simulink model "missile_simulink"  (R2025a)
settings: Solver=ode4  StartTime=0.0  StopTime=300  FixedStep=0.01  RelTol=1e-3
values from neighbouring files (symbols this model uses):
  ka = 4.5    [missile_sim.m]
  kd = 1.1    [missile_sim.m]
  ki = 14.3    [missile_sim.m]
  kr = -0.37    [missile_sim.m]
  l_m0 = 40 * d2r    (= 0.698131700798)    [missile_sim.m]
  l_t0 = -2.5 * d2r    (= -0.0436332312999)    [missile_sim.m]
  v_t = 1000    [missile_sim.m]
  x_m0 = 2000    [missile_sim.m]
  x_t0 = 100    [missile_sim.m]
  z_m0 = 0    [missile_sim.m]
  z_t0 = 20000    [missile_sim.m]
libraries: simulink x1
settings Model: Creator=jWmma  LastModifiedBy=jWmma
settings DebuggingCC: SolverPrmCheckMsg=warning

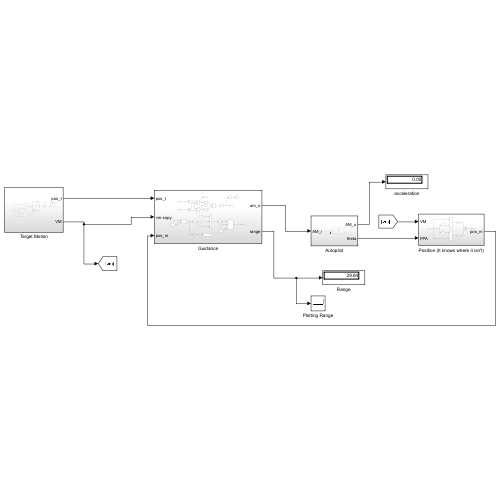
[thumbnail: Simulink's stored preview of the top-level diagram]
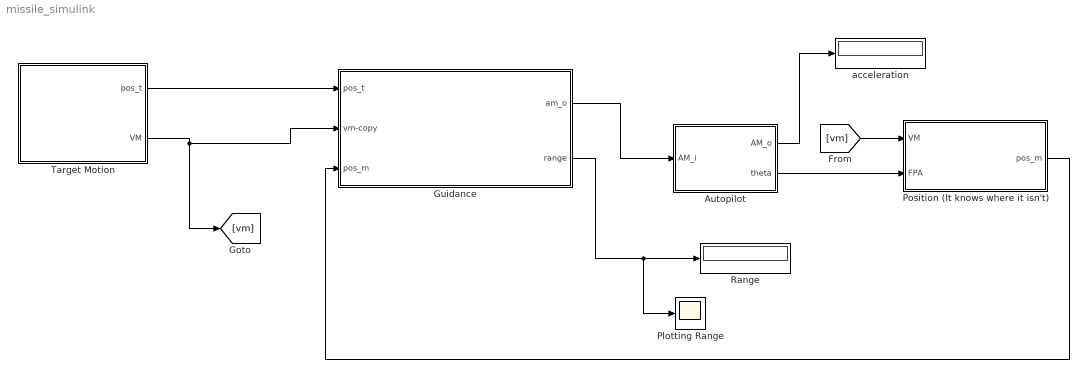
== system missile_simulink ==
  Autopilot : Subsystem
  Guidance : Subsystem
  Plotting Range : Scope
      settings: ActiveDisplayYMinimum=-88.233832620361682  ActiveDisplayYMaximum=93.627607111777422
  Position (It knows where it isn't) : Subsystem
  Range : Display
      settings: Format=bank
  Target Motion : Subsystem
  acceleration : Display
      settings: Format=bank
  wires:
  Guidance/1(am_o) -> Autopilot/1(AM_i)
  Guidance/2(range) -> Plotting Range/1, Range/1
  Autopilot/2(theta) -> Position (It knows where it isn't)/2(FPA)
  Position (It knows where it isn't)/1(pos_m) -> Guidance/3(pos_m)
  Target Motion/1(pos_t) -> Guidance/1(pos_t)
  Target Motion/2(VM) -> [vm], Guidance/2(vm-copy)
  Autopilot/1(AM_o) -> acceleration/1
  [vm] -> Position (It knows where it isn't)/1(VM)

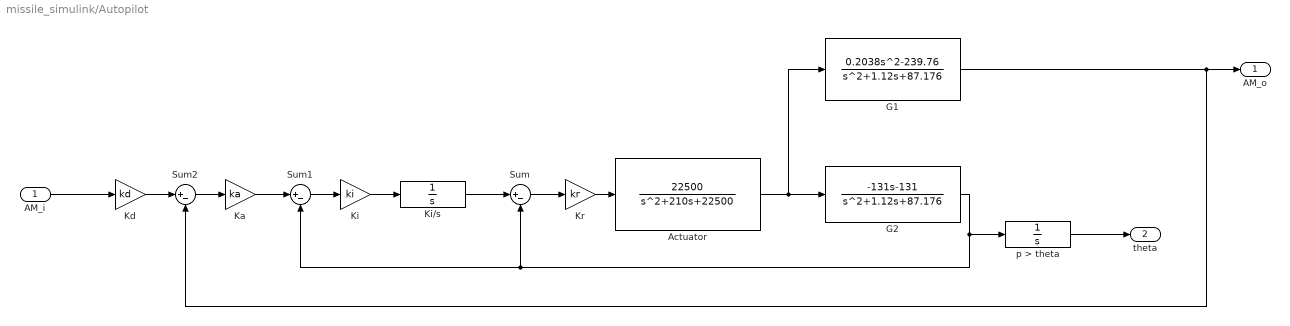
== system missile_simulink/Autopilot ==
  AM_i : Inport
  Actuator : TransferFcn  Numerator=[22500]  Denominator=[1 210 22500]
  G1 : TransferFcn  Numerator=[0.2038 0 -239.76]  Denominator=[1 1.12 87.176]
  G2 : TransferFcn  Numerator=[-131 -131]  Denominator=[1 1.12 87.176]
  Ka : Gain  Gain=ka
  Kd : Gain  Gain=kd
  Ki : Gain  Gain=ki
  Ki/s : Integrator
  Kr : Gain  Gain=kr
  Sum : Sum  Inputs=|+-
  Sum1 : Sum  Inputs=|+-
  Sum2 : Sum  Inputs=|+-
  p > theta : Integrator  InitialCondition=l_m0
  AM_o : Outport
  theta : Outport  Port=2
  wires:
  p > theta/1 -> theta/1
  Sum2/1 -> Ka/1
  G2/1 -> p > theta/1, Sum1/2, Sum/2
  AM_i/1 -> Kd/1
  Actuator/1 -> G1/1, G2/1
  Kr/1 -> Actuator/1
  Ka/1 -> Sum1/1
  Sum1/1 -> Ki/1
  Sum/1 -> Kr/1
  G1/1 -> AM_o/1, Sum2/2
  Ki/1 -> Ki/s/1
  Ki/s/1 -> Sum/1
  Kd/1 -> Sum2/1

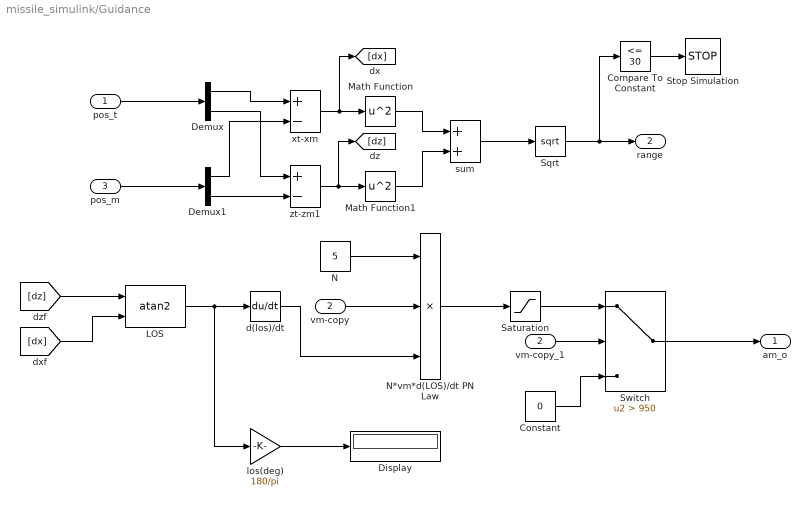
== system missile_simulink/Guidance ==
  pos_t : Inport
  vm-copy : Inport  Port=2
  pos_m : Inport  Port=3
  Compare To Constant : simulink/Logic and Bit Operations/Compare To Constant  relop=<=  const=30  OutDataTypeStr=boolean
  Constant : Constant  Value=0
  Demux : Demux  Outputs=2
  Demux1 : Demux  Outputs=2
  Display : Display
  LOS : Trigonometry  Operator=atan2
  Math Function : Math  Operator=square  OutputSignalType=real
  Math Function1 : Math  Operator=square  OutputSignalType=real
  N : Constant  Value=5
  N*vm*d(LOS)/dt PN Law : Product  Inputs=3
  Saturation : Saturate  UpperLimit=0  LowerLimit=-0.1
  Sqrt : Sqrt
  Stop Simulation : Stop
  Switch : Switch  Criteria=u2 > Threshold  Threshold=950  SaturateOnIntegerOverflow=off  InputSameDT=off
  d(los)/dt : Derivative
  los(deg) : Gain  Gain=180/pi
  sum : Sum
  vm-copy_1 : InportShadow  Port=2
  xt-xm : Sum  Inputs=+-
  zt-zm1 : Sum  Inputs=+-
  am_o : Outport
  range : Outport  Port=2
  wires:
  Math Function1/1 -> sum/2
  Demux1/2 -> zt-zm1/2
  N/1 -> N*vm*d(LOS)/dt PN Law/1
  vm-copy_1/1 -> Switch/2
  xt-xm/1 -> [dx], Math Function/1
  LOS/1 -> los(deg)/1, d(los)/dt/1
  Demux/2 -> zt-zm1/1
  zt-zm1/1 -> [dz], Math Function1/1
  Demux1/1 -> xt-xm/2
  [dx] -> LOS/2
  [dz] -> LOS/1
  los(deg)/1 -> Display/1
  pos_t/1 -> Demux/1
  Math Function/1 -> sum/1
  Sqrt/1 -> Compare To Constant/1, range/1
  vm-copy/1 -> N*vm*d(LOS)/dt PN Law/2
  pos_m/1 -> Demux1/1
  Demux/1 -> xt-xm/1
  sum/1 -> Sqrt/1
  Constant/1 -> Switch/3
  N*vm*d(LOS)/dt PN Law/1 -> Saturation/1
  d(los)/dt/1 -> N*vm*d(LOS)/dt PN Law/3
  Saturation/1 -> Switch/1
  Switch/1 -> am_o/1
  Compare To Constant/1 -> Stop Simulation/1

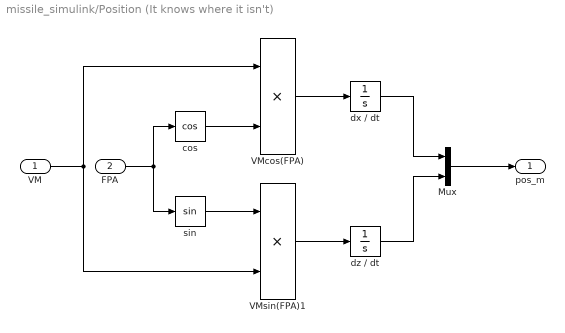
== system missile_simulink/Position (It knows where it isn't) ==
  VM : Inport
  FPA : Inport  Port=2
  Mux : Mux  Inputs=2
  VMcos(FPA) : Product
  VMsin(FPA)1 : Product
  cos : Trigonometry  Operator=cos
  dx / dt : Integrator  InitialCondition=x_m0
  dz / dt : Integrator  InitialCondition=z_m0
  sin : Trigonometry
  pos_m : Outport
  wires:
  VMsin(FPA)1/1 -> dz / dt/1
  VMcos(FPA)/1 -> dx / dt/1
  VM/1 -> VMsin(FPA)1/2, VMcos(FPA)/1
  Mux/1 -> pos_m/1
  dz / dt/1 -> Mux/2
  dx / dt/1 -> Mux/1
  sin/1 -> VMsin(FPA)1/1
  FPA/1 -> sin/1, cos/1
  cos/1 -> VMcos(FPA)/2

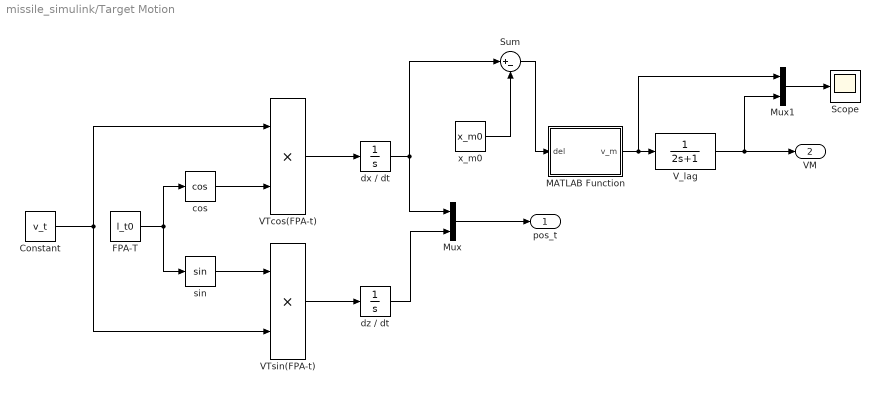
== system missile_simulink/Target Motion ==
  Constant : Constant  Value=v_t
  FPA-T : Constant  Value=l_t0
  MATLAB Function : MATLAB Function  TreatAsAtomicUnit=on
  Mux : Mux  Inputs=2
  Mux1 : Mux  Inputs=2
  Scope : Scope
      settings: ActiveDisplayYMinimum=-21.521564188528686  ActiveDisplayYMaximum=17.383580610924632
  Sum : Sum  Inputs=|+-
  VTcos(FPA-t) : Product
  VTsin(FPA-t) : Product
  V_lag : TransferFcn  Denominator=[2 1]
  cos : Trigonometry  Operator=cos
  dx / dt : Integrator  InitialCondition=x_t0
  dz / dt : Integrator  InitialCondition=z_t0
  sin : Trigonometry
  x_m0 : Constant  Value=x_m0
  pos_t : Outport
  VM : Outport  Port=2
  wires:
  VTcos(FPA-t)/1 -> dx / dt/1
  FPA-T/1 -> sin/1, cos/1
  Mux/1 -> pos_t/1
  Constant/1 -> VTsin(FPA-t)/2, VTcos(FPA-t)/1
  cos/1 -> VTcos(FPA-t)/2
  dz / dt/1 -> Mux/2
  dx / dt/1 -> Sum/1, Mux/1
  V_lag/1 -> VM/1, Mux1/2
  Sum/1 -> MATLAB Function/1(del)
  sin/1 -> VTsin(FPA-t)/1
  VTsin(FPA-t)/1 -> dz / dt/1
  MATLAB Function/1(v_m) -> Mux1/1, V_lag/1
  Mux1/1 -> Scope/1
  x_m0/1 -> Sum/2

== matlab function missile_simulink/Target Motion/MATLAB Function ==
  settings: updateMethod=DISCRETE
  data: del input; v_m output
function v_m = fcn(del)

persistent f
persistent Vel

if isempty(f)
    f = 0;
end

if isempty(Vel)
    Vel = 0;
end

if f == 0 && del > -200
    f = 1;
    Vel = 1021;
end

v_m = Vel;
